simulink model "Demo_DSRC_BSM_I_and_II_Message_cs"  (Simulink 7.6)
settings: Solver=ode5  SolverMode=SingleTasking  StartTime=0.0  StopTime=40  FixedStep=1/20  RelTol=1e-3
PreLoadFcn:
  | check_NUTS_defined;
  | 
  | assignin('base',['model_closed_' bdroot],false);
InitFcn:
  | PreScanExperimentInitFcn(bdroot)
StopFcn:
  | PreScanExperimentStopFcn(bdroot)
libraries: simulink x9, PreScanSimulinkLibrary x8, PreScanUsefulBlocks x5, simulink_extras x1
(part 3 of 3)

== system Demo_DSRC_BSM_I_and_II_Message_cs/Mazda_RX8_1/Radius and confidence computation/Limitations ==
  note: Values of radius and center point
      |   coordinates on a straight path segment
  R : Inport
  d_Phi : Inport  Port=2
  "[xp,yp]" : Inport  Port=3
  Compare To Constant : simulink/Logic and Bit Operations/Compare To Constant  SystemSampleTime=-1  relop=<=  const=K_PPPATHISSTRAIGHT_M  LogicOutDataTypeMode=boolean  ZeroCross=off
  Compare To Zero : simulink/Logic and Bit Operations/Compare To Zero  SystemSampleTime=-1  relop=~=  LogicOutDataTypeMode=boolean  ZeroCross=off
  Compare To Zero1 : simulink/Logic and Bit Operations/Compare To Zero  SystemSampleTime=-1  relop=>  LogicOutDataTypeMode=boolean  ZeroCross=off
  Constant : Constant  Value=K_PPPATHISSTRAIGHT_M
  Constant1 : Constant  Value=[0;0]
  Logical Operator : Logic  Inputs=3  AllPortsSameDT=off  OutDataTypeStr=boolean  SampleTime=GPS_sample_time
  Switch1 : Switch  Criteria=u2 > Threshold  Threshold=0.5  SampleTime=GPS_sample_time
  Switch2 : Switch  Criteria=u2 > Threshold  Threshold=0.5  SampleTime=GPS_sample_time
  Radius [m] : Outport
  Center point : Outport  Port=2
  wires:
  R/1 -> Compare To Constant/1, Switch1/1, Compare To Zero1/1
  Compare To Zero/1 -> Logical Operator/1
  Compare To Constant/1 -> Logical Operator/2
  Logical Operator/1 -> Switch1/2, Switch2/2
  Constant/1 -> Switch1/3
  "[xp,yp]"/1 -> Switch2/1
  Constant1/1 -> Switch2/3
  Switch2/1 -> Center point/1
  Switch1/1 -> Radius [m]/1
  Compare To Zero1/1 -> Logical Operator/3
  d_Phi/1 -> Compare To Zero/1

== system Demo_DSRC_BSM_I_and_II_Message_cs/Mazda_RX8_1/Radius and confidence computation/Previous reading ==
  note: Determines previous value of signals
  Lat_in [deg] : Inport
  Long_in [deg] : Inport  Port=2
  Heading_in [deg] : Inport  Port=3
  Alt_in [m] : Inport  Port=4
  Demux : Demux
  Mux : Mux
  Unit Delay : UnitDelay  SampleTime=-1
  Lat2 [deg] : Outport
  Long2 [deg] : Outport  Port=2
  Heading2 [deg] : Outport  Port=3
  Alt2 [m] : Outport  Port=4
  wires:
  Lat_in [deg]/1 -> Mux/1
  Long_in [deg]/1 -> Mux/2
  Mux/1 -> Unit Delay/1
  Unit Delay/1 -> Demux/1
  Demux/1 -> Lat2 [deg]/1
  Demux/2 -> Long2 [deg]/1
  Heading_in [deg]/1 -> Mux/3
  Alt_in [m]/1 -> Mux/4
  Demux/3 -> Heading2 [deg]/1
  Demux/4 -> Alt2 [m]/1

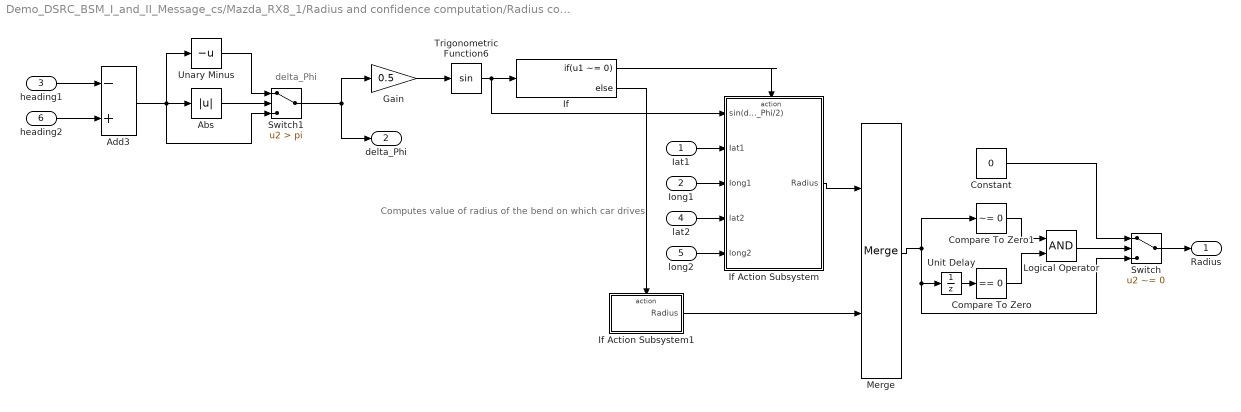
== system Demo_DSRC_BSM_I_and_II_Message_cs/Mazda_RX8_1/Radius and confidence computation/Radius computation ==
  note: delta_Phi
  note: Computes value of radius
      |    of the bend on which car drives
  Iat1 : Inport
  Iong1 : Inport  Port=2
  heading1 : Inport  Port=3
  lat2 : Inport  Port=4
  long2 : Inport  Port=5
  heading2 : Inport  Port=6
  Abs : Abs
  Add3 : Sum  Inputs=-+
  Compare To Zero : simulink/Logic and Bit Operations/Compare To Zero  SystemSampleTime=-1  relop===  LogicOutDataTypeMode=boolean  ZeroCross=off
  Compare To Zero1 : simulink/Logic and Bit Operations/Compare To Zero  SystemSampleTime=-1  relop=~=  LogicOutDataTypeMode=boolean  ZeroCross=off
  Constant : Constant  Value=0
  Gain : Gain  Gain=0.5
  If : If  IfExpression=u1 ~= 0
  If Action Subsystem : Subsystem  TreatAsAtomicUnit=on
  If Action Subsystem1 : Subsystem  TreatAsAtomicUnit=on
  Logical Operator : Logic  AllPortsSameDT=off  OutDataTypeStr=boolean
  Merge : Merge
  Switch : Switch  Criteria=u2 ~= 0  SampleTime=GPS_sample_time
  Switch1 : Switch  Criteria=u2 > Threshold  Threshold=pi
  Trigonometric Function6 : Trigonometry
  Unary Minus : UnaryMinus
  Unit Delay : UnitDelay  SampleTime=-1
  Radius : Outport
  delta_Phi : Outport  Port=2
  wires:
  Gain/1 -> Trigonometric Function6/1
  Trigonometric Function6/1 -> If/1, If Action Subsystem/1(sin(delta_Phi/2))
  If/1 -> If Action Subsystem/Action
  If/2 -> If Action Subsystem1/Action
  If Action Subsystem/1(Radius) -> Merge/1
  If Action Subsystem1/1(Radius) -> Merge/2
  Merge/1 -> Compare To Zero1/1, Unit Delay/1, Switch/3
  Unit Delay/1 -> Compare To Zero/1
  Compare To Zero1/1 -> Logical Operator/1
  Compare To Zero/1 -> Logical Operator/2
  Logical Operator/1 -> Switch/2
  Constant/1 -> Switch/1
  Switch/1 -> Radius/1
  heading1/1 -> Add3/1
  heading2/1 -> Add3/2
  Add3/1 -> Abs/1, Switch1/3, Unary Minus/1
  Abs/1 -> Switch1/2
  Unary Minus/1 -> Switch1/1
  Switch1/1 -> Gain/1, delta_Phi/1
  Iat1/1 -> If Action Subsystem/2(Iat1)
  Iong1/1 -> If Action Subsystem/3(Iong1)
  lat2/1 -> If Action Subsystem/4(lat2)
  long2/1 -> If Action Subsystem/5(long2)

== system Demo_DSRC_BSM_I_and_II_Message_cs/Mazda_RX8_1/Radius and confidence computation/Rate transition ==
  note: Changes rate transition of
      |    signals to GPS sampling rate
  Lat_in [deg] : Inport
  Long_in [deg] : Inport  Port=2
  Alt_in [m] : Inport  Port=3
  Heading_in [deg] : Inport  Port=4
  Demux : Demux
  Mux : Mux
  Rate Transition : RateTransition  Integrity=off  OutPortSampleTime=GPS_sample_time
  Lat [deg] : Outport
  Long [deg] : Outport  Port=2
  Heading [deg] : Outport  Port=3
  Alt [m] : Outport  Port=4
  wires:
  Lat_in [deg]/1 -> Mux/1
  Long_in [deg]/1 -> Mux/2
  Alt_in [m]/1 -> Mux/3
  Heading_in [deg]/1 -> Mux/4
  Mux/1 -> Rate Transition/1
  Rate Transition/1 -> Demux/1
  Demux/1 -> Lat [deg]/1
  Demux/2 -> Long [deg]/1
  Demux/3 -> Alt [m]/1
  Demux/4 -> Heading [deg]/1

== system Demo_DSRC_BSM_I_and_II_Message_cs/Mazda_RX8_1/SELF_Demux/compas converter ==
  rotz [rad] : Inport
  cart2compas : Subsystem
  rad2deg : Gain  Gain=180/pi
  heading [deg] : Outport
  wires:
  cart2compas/1(heading [deg]) -> heading [deg]/1
  rotz [rad]/1 -> rad2deg/1
  rad2deg/1 -> cart2compas/1(Angle [deg])

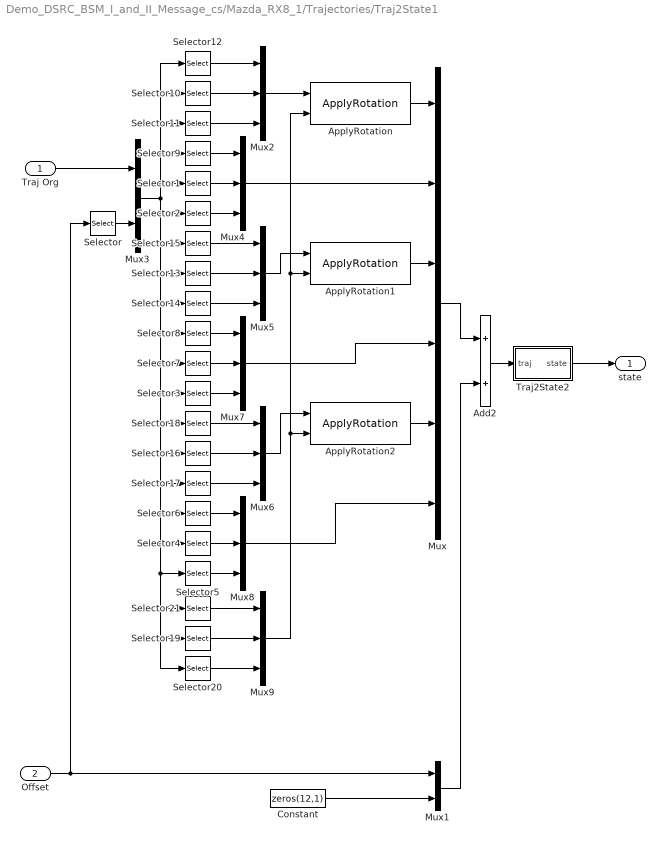
== system Demo_DSRC_BSM_I_and_II_Message_cs/Mazda_RX8_1/Trajectories/Traj2State1 ==
  Traj Org : Inport
  Offset : Inport  Port=2
  Add2 : Sum
  ApplyRotation : PreScanSimulinkLibrary/ApplyRotation  SystemSampleTime=-1
  ApplyRotation1 : PreScanSimulinkLibrary/ApplyRotation  SystemSampleTime=-1
  ApplyRotation2 : PreScanSimulinkLibrary/ApplyRotation  SystemSampleTime=-1
  Constant : Constant  Value=zeros(12,1)
  Mux : Mux  Inputs=6
  Mux1 : Mux  Inputs=2
  Mux{2,4..9} (7 alike) : Mux  Inputs=3
  Mux3 : Mux  Inputs=2
  Selector : Selector  InputPortWidth=6  IndexOptions=Index vector (dialog)  Indices=[4 5 6]  OutputSizes=1
  Selector1 : Selector  InputPortWidth=21  IndexOptions=Index vector (dialog)  Indices=[5]  OutputSizes=1
  Selector10 : Selector  InputPortWidth=21  IndexOptions=Index vector (dialog)  Indices=[2]  OutputSizes=1
  Selector11 : Selector  InputPortWidth=21  IndexOptions=Index vector (dialog)  Indices=[3]  OutputSizes=1
  Selector12 : Selector  InputPortWidth=21  IndexOptions=Index vector (dialog)  Indices=[1]  OutputSizes=1
  Selector13 : Selector  InputPortWidth=21  IndexOptions=Index vector (dialog)  Indices=[8]  OutputSizes=1
  Selector14 : Selector  InputPortWidth=21  IndexOptions=Index vector (dialog)  Indices=[9]  OutputSizes=1
  Selector15 : Selector  InputPortWidth=21  IndexOptions=Index vector (dialog)  Indices=[7]  OutputSizes=1
  Selector16 : Selector  InputPortWidth=21  IndexOptions=Index vector (dialog)  Indices=[14]  OutputSizes=1
  Selector17 : Selector  InputPortWidth=21  IndexOptions=Index vector (dialog)  Indices=[15]  OutputSizes=1
  Selector18 : Selector  InputPortWidth=21  IndexOptions=Index vector (dialog)  Indices=[13]  OutputSizes=1
  Selector19 : Selector  InputPortWidth=21  IndexOptions=Index vector (dialog)  Indices=[20]  OutputSizes=1
  Selector2 : Selector  InputPortWidth=21  IndexOptions=Index vector (dialog)  Indices=[6]  OutputSizes=1
  Selector20 : Selector  InputPortWidth=21  IndexOptions=Index vector (dialog)  Indices=[21]  OutputSizes=1
  Selector21 : Selector  InputPortWidth=21  IndexOptions=Index vector (dialog)  Indices=[19]  OutputSizes=1
  Selector3 : Selector  InputPortWidth=21  IndexOptions=Index vector (dialog)  Indices=[12]  OutputSizes=1
  Selector4 : Selector  InputPortWidth=21  IndexOptions=Index vector (dialog)  Indices=[17]  OutputSizes=1
  Selector5 : Selector  InputPortWidth=21  IndexOptions=Index vector (dialog)  Indices=[18]  OutputSizes=1
  Selector6 : Selector  InputPortWidth=21  IndexOptions=Index vector (dialog)  Indices=[16]  OutputSizes=1
  Selector7 : Selector  InputPortWidth=21  IndexOptions=Index vector (dialog)  Indices=[11]  OutputSizes=1
  Selector8 : Selector  InputPortWidth=21  IndexOptions=Index vector (dialog)  Indices=[10]  OutputSizes=1
  Selector9 : Selector  InputPortWidth=21  IndexOptions=Index vector (dialog)  Indices=[4]  OutputSizes=1
  Traj2State2 : Subsystem
  state : Outport
  wires:
  Mux9/1 -> ApplyRotation2/2, ApplyRotation1/2, ApplyRotation/2
  Selector20/1 -> Mux9/3
  Selector19/1 -> Mux9/2
  Selector21/1 -> Mux9/1
  Selector5/1 -> Mux8/3
  Selector4/1 -> Mux8/2
  Selector6/1 -> Mux8/1
  Mux8/1 -> Mux/6
  Mux6/1 -> ApplyRotation2/1
  Mux7/1 -> Mux/4
  ApplyRotation2/1 -> Mux/5
  Selector3/1 -> Mux7/3
  Selector7/1 -> Mux7/2
  Selector8/1 -> Mux7/1
  Mux4/1 -> Mux/2
  Mux5/1 -> ApplyRotation1/1
  ApplyRotation1/1 -> Mux/3
  Mux2/1 -> ApplyRotation/1
  ApplyRotation/1 -> Mux/1
  Selector2/1 -> Mux4/3
  Selector1/1 -> Mux4/2
  Selector9/1 -> Mux4/1
  Selector17/1 -> Mux6/3
  Selector16/1 -> Mux6/2
  Selector18/1 -> Mux6/1
  Selector14/1 -> Mux5/3
  Selector13/1 -> Mux5/2
  Selector15/1 -> Mux5/1
  Selector11/1 -> Mux2/3
  Selector10/1 -> Mux2/2
  Selector12/1 -> Mux2/1
  Mux3/1 -> Selector8/1, Selector7/1, Selector3/1, Selector18/1, Selector16/1, Selector17/1, Selector6/1, Selector20/1, Selector19/1, Selector21/1, Selector5/1, Selector4/1, Selector14/1, Selector13/1, Selector15/1, Selector2/1, Selector1/1, Selector9/1, Selector12/1, Selector10/1, Selector11/1
  Mux1/1 -> Add2/2
  Constant/1 -> Mux1/2
  Add2/1 -> Traj2State2/1(traj)
  Selector/1 -> Mux3/2
  Traj Org/1 -> Mux3/1
  Offset/1 -> Mux1/1, Selector/1
  Mux/1 -> Add2/1
  Traj2State2/1(state) -> state/1

== system Demo_DSRC_BSM_I_and_II_Message_cs/Mazda_RX8_1/Trajectories/Trajectory_1 ==
  From Workspace : FromWorkspace  VariableName=trajectory  SampleTime=TimeStep  OutputAfterFinalValue=Holding final value
  From Workspace1 : FromWorkspace  VariableName=trajectory  SampleTime=TimeStep  OutputAfterFinalValue=Setting to zero
  Mux : Mux  Inputs=2
  Selector1 : Selector  InputPortWidth=24  IndexOptions=Index vector (dialog)  Indices=[7:18]  OutputSizes=1
  Selector9 : Selector  InputPortWidth=24  IndexOptions=Index vector (dialog)  Indices=[1:6]  OutputSizes=1
  trajectory : Outport
  wires:
  Selector1/1 -> Mux/2
  Selector9/1 -> Mux/1
  Mux/1 -> trajectory/1
  From Workspace1/1 -> Selector1/1
  From Workspace/1 -> Selector9/1

== system Demo_DSRC_BSM_I_and_II_Message_cs/Ford_Fiesta_1/DSRC Receiver BSM I and II/DSRC_Rx_Demux/Reorder ==
  In : Inport
  Selector1 : Selector  InputPortWidth=InputPortWidth  IndexOptions=Index vector (dialog)  Indices=Elements  OutputSizes=1
  Out : Outport
  wires:
  In/1 -> Selector1/1
  Selector1/1 -> Out/1

== system Demo_DSRC_BSM_I_and_II_Message_cs/Ford_Fiesta_1/DSRC Receiver BSM I and II/DSRC_Rx_Demux/compas converter ==
  rotz [rad] : Inport
  cart2compas : Subsystem
  rad2deg : Gain  Gain=180/pi
  heading [deg] : Outport
  wires:
  cart2compas/1(heading [deg]) -> heading [deg]/1
  rotz [rad]/1 -> rad2deg/1
  rad2deg/1 -> cart2compas/1(Angle [deg])

== system Demo_DSRC_BSM_I_and_II_Message_cs/Ford_Fiesta_1/SELF_Demux/compas converter/cart2compas ==
  Angle [deg] : Inport
  Constant : Constant  Value=90
  Constant1 : Constant  Value=360
  Gain : Gain  Gain=1/360
  Gain1 : Gain  Gain=360
  Gain2 : Gain  Gain=-1
  Rounding Function : Rounding
  Sum : Sum  Inputs=|-+
  Sum1 : Sum  Inputs=-+|
  Sum2 : Sum  Inputs=++|
  heading [deg] : Outport
  wires:
  Sum2/1 -> heading [deg]/1
  Constant1/1 -> Sum2/1
  Gain2/1 -> Sum2/2
  Constant/1 -> Sum1/1
  Sum1/1 -> Sum/2, Gain/1
  Sum/1 -> Gain2/1
  Angle [deg]/1 -> Sum1/2
  Gain1/1 -> Sum/1
  Rounding Function/1 -> Gain1/1
  Gain/1 -> Rounding Function/1

== system Demo_DSRC_BSM_I_and_II_Message_cs/Ford_Fiesta_1/Trajectories/Traj2State1/Traj2State2 ==
  traj : Inport
  MuxState : Subsystem
  Traj2MuxState_Ext : Subsystem
  state : Outport
  wires:
  Traj2MuxState_Ext/9(Y [rad]) -> MuxState/9(Y [rad])
  Traj2MuxState_Ext/8(P [rad]) -> MuxState/8(P [rad])
  Traj2MuxState_Ext/7(R [rad]) -> MuxState/7(R [rad])
  Traj2MuxState_Ext/6(dz [m/s]) -> MuxState/6(dz [m/s])
  Traj2MuxState_Ext/5(dy [m/s]) -> MuxState/5(dy [m/s])
  Traj2MuxState_Ext/4(dx [m/s]) -> MuxState/4(dx [m/s])
  Traj2MuxState_Ext/3(z [m]) -> MuxState/3(z [m])
  Traj2MuxState_Ext/2(y [m]) -> MuxState/2(y [m])
  Traj2MuxState_Ext/1(x [m]) -> MuxState/1(x [m])
  MuxState/1(state) -> state/1
  traj/1 -> Traj2MuxState_Ext/1(Traj)

== system Demo_DSRC_BSM_I_and_II_Message_cs/Mazda_RX8_1/Basic Safety Message II/Enabled Basic Safety Message I and II/Enabled Confidence ==
  In1 : Inport
  Enable : EnablePort  PropagateVarSize=During execution
  Out1 : Outport  OutputWhenDisabled=reset  InitialOutput=0
  wires:
  In1/1 -> Out1/1

== system Demo_DSRC_BSM_I_and_II_Message_cs/Mazda_RX8_1/Basic Safety Message II/Enabled Basic Safety Message I and II/Enabled Eventflag ==
  In1 : Inport
  Enable : EnablePort  PropagateVarSize=During execution
  Out1 : Outport  OutputWhenDisabled=reset  InitialOutput=0
  wires:
  In1/1 -> Out1/1

== system Demo_DSRC_BSM_I_and_II_Message_cs/Mazda_RX8_1/Basic Safety Message II/Enabled Basic Safety Message I and II/Enabled Exterior lights ==
  In1 : Inport
  Enable : EnablePort  PropagateVarSize=During execution
  Out1 : Outport  OutputWhenDisabled=reset  InitialOutput=0
  wires:
  In1/1 -> Out1/1

== system Demo_DSRC_BSM_I_and_II_Message_cs/Mazda_RX8_1/Basic Safety Message II/Enabled Basic Safety Message I and II/Enabled itemCnt ==
  In1 : Inport
  Enable : EnablePort  PropagateVarSize=During execution
  Out1 : Outport  OutputWhenDisabled=reset  InitialOutput=0
  wires:
  In1/1 -> Out1/1

== system Demo_DSRC_BSM_I_and_II_Message_cs/Mazda_RX8_1/Basic Safety Message II/Enabled Basic Safety Message I and II/Enabled radiusOfCurve ==
  In1 : Inport
  Enable : EnablePort  PropagateVarSize=During execution
  Out1 : Outport  OutputWhenDisabled=reset  InitialOutput=0
  wires:
  In1/1 -> Out1/1

== system Demo_DSRC_BSM_I_and_II_Message_cs/Mazda_RX8_1/Basic Safety Message II/Enabled Basic Safety Message I and II/Enabled Throttle position ==
  In1 : Inport
  Enable : EnablePort  PropagateVarSize=During execution
  Out1 : Outport  OutputWhenDisabled=reset  InitialOutput=0
  wires:
  In1/1 -> Out1/1

== system Demo_DSRC_BSM_I_and_II_Message_cs/Mazda_RX8_1/Basic Safety Message II/Enabled Basic Safety Message I and II/Enabled path history ==
  In1 : Inport
  Enable : EnablePort  PropagateVarSize=During execution
  Out1 : Outport  OutputWhenDisabled=reset  InitialOutput=0
  wires:
  In1/1 -> Out1/1

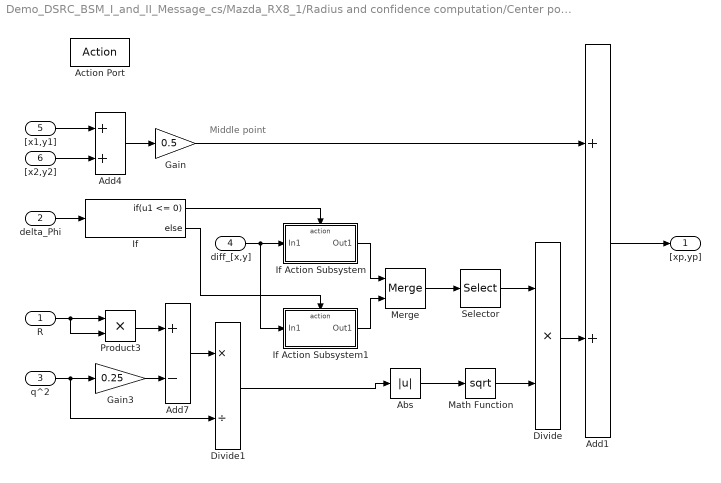
== system Demo_DSRC_BSM_I_and_II_Message_cs/Mazda_RX8_1/Radius and confidence computation/Center point of the bend/If Action Subsystem ==
  note: Middle point
  R : Inport
  delta_Phi : Inport  Port=2
  q^2 : Inport  Port=3
  diff_[x,y] : Inport  Port=4
  "[x1,y1]" : Inport  Port=5
  "[x2,y2]" : Inport  Port=6
  Action Port : ActionPort  PropagateVarSize=During execution  ActionType=then
  Abs : Abs
  Add1 : Sum
  Add4 : Sum
  Add7 : Sum  Inputs=+-
  Divide : Product  Inputs=**
  Divide1 : Product  Inputs=*/
  Gain : Gain  Gain=0.5
  Gain3 : Gain  Gain=0.25
  If : If  IfExpression=u1 <= 0
  If Action Subsystem : Subsystem  TreatAsAtomicUnit=on
  If Action Subsystem1 : Subsystem  TreatAsAtomicUnit=on
  Math Function : Math  Operator=sqrt  SaturateOnIntegerOverflow=on
  Merge : Merge
  Product3 : Product  RndMeth=Zero
  Selector : Selector  InputPortWidth=2  IndexOptions=Index vector (dialog)  Indices=[2 1]  OutputSizes=1
  "[xp,yp]" : Outport  InitialOutput=0
  wires:
  Add4/1 -> Gain/1
  "[x1,y1]"/1 -> Add4/1
  "[x2,y2]"/1 -> Add4/2
  delta_Phi/1 -> If/1
  If/1 -> If Action Subsystem/Action
  If/2 -> If Action Subsystem1/Action
  diff_[x,y]/1 -> If Action Subsystem/1(In1), If Action Subsystem1/1(In1)
  Gain3/1 -> Add7/2
  Product3/1 -> Add7/1
  Math Function/1 -> Divide/2
  If Action Subsystem/1(Out1) -> Merge/1
  If Action Subsystem1/1(Out1) -> Merge/2
  Merge/1 -> Selector/1
  q^2/1 -> Gain3/1, Divide1/2
  Selector/1 -> Divide/1
  Add1/1 -> "[xp,yp]"/1
  Divide/1 -> Add1/2
  Add7/1 -> Divide1/1
  Divide1/1 -> Abs/1
  R/1 -> Product3/1, Product3/2
  Gain/1 -> Add1/1
  Abs/1 -> Math Function/1

== system Demo_DSRC_BSM_I_and_II_Message_cs/Mazda_RX8_1/Radius and confidence computation/Center point of the bend/If Action Subsystem1 ==
  Action Port : ActionPort  PropagateVarSize=During execution  ActionType=else
  Constant : Constant  Value=zeros(2,1)
  "[xp,yp]" : Outport  InitialOutput=0
  wires:
  Constant/1 -> "[xp,yp]"/1

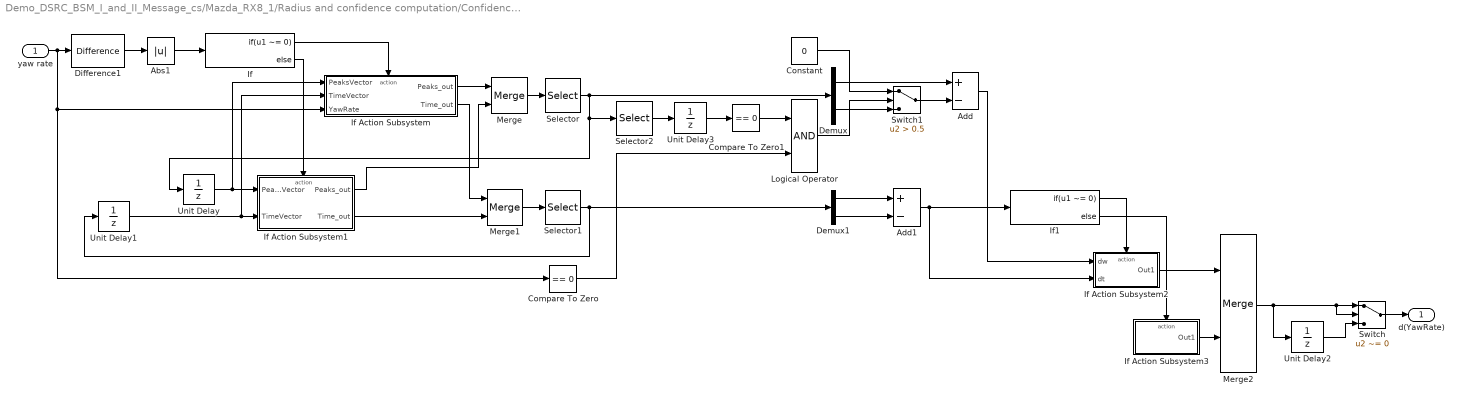
== system Demo_DSRC_BSM_I_and_II_Message_cs/Mazda_RX8_1/Radius and confidence computation/Confidence level/Derivative approximation ==
  yaw rate : Inport
  Abs1 : Abs
  Add : Sum  Inputs=+-
  Add1 : Sum  Inputs=+-
  Compare To Zero : simulink/Logic and Bit Operations/Compare To Zero  SystemSampleTime=-1  relop===  LogicOutDataTypeMode=uint8
  Compare To Zero1 : simulink/Logic and Bit Operations/Compare To Zero  SystemSampleTime=-1  relop===  LogicOutDataTypeMode=uint8
  Constant : Constant  Value=0
  Demux : Demux  Outputs=2
  Demux1 : Demux  Outputs=2
  Difference1 : simulink/Discrete/Difference  SystemSampleTime=-1  ICPrevInput=0.0  OutMin=[]  OutMax=[]  OutDataType=fixdt(1, 16)  OutScaling=2^-10  DoSatur=off
  If : If  IfExpression=u1 ~= 0
  If Action Subsystem : Subsystem  TreatAsAtomicUnit=on
  If Action Subsystem1 : Subsystem  TreatAsAtomicUnit=on
  If Action Subsystem2 : Subsystem  TreatAsAtomicUnit=on
  If Action Subsystem3 : Subsystem  TreatAsAtomicUnit=on
  If1 : If  IfExpression=u1 ~= 0
  Logical Operator : Logic  AllPortsSameDT=off  OutDataTypeStr=boolean
  Merge : Merge  InitialOutput=0
  Merge1 : Merge  InitialOutput=0
  Merge2 : Merge  InitialOutput=0
  Selector : Selector  InputPortWidth=3  IndexOptions=Index vector (dialog)  Indices=[1 2]  OutputSizes=1
  Selector1 : Selector  InputPortWidth=3  IndexOptions=Index vector (dialog)  Indices=[1 2]  OutputSizes=1
  Selector2 : Selector  InputPortWidth=2  IndexOptions=Index vector (dialog)  Indices=1  OutputSizes=1
  Switch : Switch  Criteria=u2 ~= 0  Threshold=1e-6
  Switch1 : Switch  Criteria=u2 > Threshold  Threshold=0.5
  Unit Delay{,1..3} (4 alike) : UnitDelay  SampleTime=-1
  d(YawRate) : Outport
  wires:
  If/1 -> If Action Subsystem/Action
  If/2 -> If Action Subsystem1/Action
  Unit Delay/1 -> If Action Subsystem1/1(PeaksVector), If Action Subsystem/1(PeaksVector)
  If Action Subsystem/1(Peaks_out) -> Merge/1
  Unit Delay1/1 -> If Action Subsystem1/2(TimeVector), If Action Subsystem/2(TimeVector)
  If Action Subsystem1/1(Peaks_out) -> Merge/2
  If Action Subsystem/2(Time_out) -> Merge1/1
  If Action Subsystem1/2(Time_out) -> Merge1/2
  Merge/1 -> Selector/1
  Merge1/1 -> Selector1/1
  Selector/1 -> Demux/1, Unit Delay/1, Selector2/1
  Selector1/1 -> Unit Delay1/1, Demux1/1
  Demux/1 -> Add/1
  Demux1/1 -> Add1/1
  Demux1/2 -> Add1/2
  Add/1 -> If Action Subsystem2/1(dw)
  Difference1/1 -> Abs1/1
  Merge2/1 -> Unit Delay2/1, Switch/1, Switch/2
  Unit Delay2/1 -> Switch/3
  Abs1/1 -> If/1
  Add1/1 -> If1/1, If Action Subsystem2/2(dt)
  If1/1 -> If Action Subsystem2/Action
  If1/2 -> If Action Subsystem3/Action
  If Action Subsystem2/1(Out1) -> Merge2/1
  If Action Subsystem3/1(Out1) -> Merge2/2
  yaw rate/1 -> Difference1/1, If Action Subsystem/3(YawRate), Compare To Zero/1
  Switch/1 -> d(YawRate)/1
  Selector2/1 -> Unit Delay3/1
  Unit Delay3/1 -> Compare To Zero1/1
  Compare To Zero1/1 -> Logical Operator/1
  Compare To Zero/1 -> Logical Operator/2
  Logical Operator/1 -> Switch1/2
  Demux/2 -> Switch1/3
  Switch1/1 -> Add/2
  Constant/1 -> Switch1/1

== system Demo_DSRC_BSM_I_and_II_Message_cs/Mazda_RX8_1/Radius and confidence computation/Confidence level/FIR filter1 ==
  In1 : Inport
  Add : Sum  Inputs=++++++++++
  Gain : Gain  Gain=0.1
  Unit Delay{1..9} (9 alike) : UnitDelay  SampleTime=-1
  Out1 : Outport
  wires:
  In1/1 -> Add/1, Unit Delay1/1
  Add/1 -> Gain/1
  Unit Delay1/1 -> Add/2, Unit Delay2/1
  Unit Delay2/1 -> Add/3, Unit Delay3/1
  Unit Delay3/1 -> Add/4, Unit Delay4/1
  Unit Delay4/1 -> Add/5, Unit Delay5/1
  Unit Delay5/1 -> Add/6, Unit Delay6/1
  Unit Delay6/1 -> Add/7, Unit Delay7/1
  Unit Delay7/1 -> Add/8, Unit Delay8/1
  Unit Delay8/1 -> Add/9, Unit Delay9/1
  Unit Delay9/1 -> Add/10
  Gain/1 -> Out1/1

== system Demo_DSRC_BSM_I_and_II_Message_cs/Mazda_RX8_1/Radius and confidence computation/Confidence level/FIR filter2 ==
  In1 : Inport
  Add : Sum  Inputs=++++++++
  Gain : Gain  Gain=1/8
  Unit Delay{1..7} (7 alike) : UnitDelay  SampleTime=-1
  Out1 : Outport
  wires:
  Unit Delay4/1 -> Add/5, Unit Delay5/1
  Unit Delay3/1 -> Unit Delay4/1, Add/4
  Unit Delay2/1 -> Unit Delay3/1, Add/3
  Unit Delay1/1 -> Unit Delay2/1, Add/2
  Add/1 -> Gain/1
  In1/1 -> Unit Delay1/1, Add/1
  Gain/1 -> Out1/1
  Unit Delay7/1 -> Add/8
  Unit Delay6/1 -> Add/7, Unit Delay7/1
  Unit Delay5/1 -> Add/6, Unit Delay6/1

== system Demo_DSRC_BSM_I_and_II_Message_cs/Mazda_RX8_1/Radius and confidence computation/Radius computation/If Action Subsystem ==
  sin(delta_Phi/2) : Inport
  Iat1 : Inport  Port=2
  Iong1 : Inport  Port=3
  lat2 : Inport  Port=4
  long2 : Inport  Port=5
  Action Port : ActionPort  PropagateVarSize=During execution  ActionType=then
  Abs : Abs
  Chord length1 : Subsystem
  Constant : Constant  Value=2
  Divide : Product  Inputs=*//
  Radius : Outport  InitialOutput=0
  wires:
  Constant/1 -> Divide/2
  Chord length1/1(chord) -> Divide/1
  sin(delta_Phi/2)/1 -> Divide/3
  Divide/1 -> Abs/1
  Abs/1 -> Radius/1
  Iong1/1 -> Chord length1/2(long1)
  long2/1 -> Chord length1/3(long2)
  Iat1/1 -> Chord length1/1(lat1)
  lat2/1 -> Chord length1/4(lat2)

== system Demo_DSRC_BSM_I_and_II_Message_cs/Mazda_RX8_1/Radius and confidence computation/Radius computation/If Action Subsystem1 ==
  Action Port : ActionPort  PropagateVarSize=During execution  ActionType=else
  Constant : Constant  Value=0
  Radius : Outport  InitialOutput=0
  wires:
  Constant/1 -> Radius/1

== system Demo_DSRC_BSM_I_and_II_Message_cs/Mazda_RX8_1/SELF_Demux/compas converter/cart2compas ==
  Angle [deg] : Inport
  Constant : Constant  Value=90
  Constant1 : Constant  Value=360
  Gain : Gain  Gain=1/360
  Gain1 : Gain  Gain=360
  Gain2 : Gain  Gain=-1
  Rounding Function : Rounding
  Sum : Sum  Inputs=|-+
  Sum1 : Sum  Inputs=-+|
  Sum2 : Sum  Inputs=++|
  heading [deg] : Outport
  wires:
  Sum2/1 -> heading [deg]/1
  Constant1/1 -> Sum2/1
  Gain2/1 -> Sum2/2
  Constant/1 -> Sum1/1
  Sum1/1 -> Sum/2, Gain/1
  Sum/1 -> Gain2/1
  Angle [deg]/1 -> Sum1/2
  Gain1/1 -> Sum/1
  Rounding Function/1 -> Gain1/1
  Gain/1 -> Rounding Function/1

== system Demo_DSRC_BSM_I_and_II_Message_cs/Mazda_RX8_1/Trajectories/Traj2State1/Traj2State2 ==
  traj : Inport
  MuxState : Subsystem
  Traj2MuxState_Ext : Subsystem
  state : Outport
  wires:
  Traj2MuxState_Ext/9(Y [rad]) -> MuxState/9(Y [rad])
  Traj2MuxState_Ext/8(P [rad]) -> MuxState/8(P [rad])
  Traj2MuxState_Ext/7(R [rad]) -> MuxState/7(R [rad])
  Traj2MuxState_Ext/6(dz [m/s]) -> MuxState/6(dz [m/s])
  Traj2MuxState_Ext/5(dy [m/s]) -> MuxState/5(dy [m/s])
  Traj2MuxState_Ext/4(dx [m/s]) -> MuxState/4(dx [m/s])
  Traj2MuxState_Ext/3(z [m]) -> MuxState/3(z [m])
  Traj2MuxState_Ext/2(y [m]) -> MuxState/2(y [m])
  Traj2MuxState_Ext/1(x [m]) -> MuxState/1(x [m])
  MuxState/1(state) -> state/1
  traj/1 -> Traj2MuxState_Ext/1(Traj)

== system Demo_DSRC_BSM_I_and_II_Message_cs/Ford_Fiesta_1/DSRC Receiver BSM I and II/DSRC_Rx_Demux/compas converter/cart2compas ==
  Angle [deg] : Inport
  Constant : Constant  Value=90
  Constant1 : Constant  Value=360
  Gain : Gain  Gain=1/360
  Gain1 : Gain  Gain=360
  Gain2 : Gain  Gain=-1
  Rounding Function : Rounding
  Sum : Sum  Inputs=|-+
  Sum1 : Sum  Inputs=-+|
  Sum2 : Sum  Inputs=++|
  heading [deg] : Outport
  wires:
  Sum2/1 -> heading [deg]/1
  Constant1/1 -> Sum2/1
  Gain2/1 -> Sum2/2
  Constant/1 -> Sum1/1
  Sum1/1 -> Sum/2, Gain/1
  Sum/1 -> Gain2/1
  Angle [deg]/1 -> Sum1/2
  Gain1/1 -> Sum/1
  Rounding Function/1 -> Gain1/1
  Gain/1 -> Rounding Function/1

== system Demo_DSRC_BSM_I_and_II_Message_cs/Ford_Fiesta_1/Trajectories/Traj2State1/Traj2State2/MuxState ==
  x [m] : Inport
  y [m] : Inport  Port=2
  z [m] : Inport  Port=3
  dx [m/s] : Inport  Port=4
  dy [m/s] : Inport  Port=5
  dz [m/s] : Inport  Port=6
  R [rad] : Inport  Port=7
  P [rad] : Inport  Port=8
  Y [rad] : Inport  Port=9
  Mux : Mux  Inputs=9
  state : Outport
  wires:
  z [m]/1 -> Mux/3
  y [m]/1 -> Mux/2
  x [m]/1 -> Mux/1
  Y [rad]/1 -> Mux/9
  P [rad]/1 -> Mux/8
  R [rad]/1 -> Mux/7
  dz [m/s]/1 -> Mux/6
  dy [m/s]/1 -> Mux/5
  dx [m/s]/1 -> Mux/4
  Mux/1 -> state/1

== system Demo_DSRC_BSM_I_and_II_Message_cs/Ford_Fiesta_1/Trajectories/Traj2State1/Traj2State2/Traj2MuxState_Ext ==
  Traj : Inport
  Terminator{1..9} (9 alike) : Terminator
  demux : Subsystem
  x [m] : Outport
  y [m] : Outport  Port=2
  z [m] : Outport  Port=3
  dx [m/s] : Outport  Port=4
  dy [m/s] : Outport  Port=5
  dz [m/s] : Outport  Port=6
  R [rad] : Outport  Port=7
  P [rad] : Outport  Port=8
  Y [rad] : Outport  Port=9
  wires:
  demux/9(Y) -> Y [rad]/1
  demux/7(R) -> R [rad]/1
  demux/5(vely) -> dy [m/s]/1
  demux/4(velx) -> dx [m/s]/1
  demux/10(velR) -> Terminator4/1
  demux/11(velP) -> Terminator5/1
  demux/12(velY) -> Terminator1/1
  demux/13(accx) -> Terminator8/1
  demux/14(accy) -> Terminator9/1
  demux/15(accz) -> Terminator7/1
  demux/18(accY) -> Terminator2/1
  demux/16(accR) -> Terminator3/1
  demux/17(accP) -> Terminator6/1
  demux/3(z) -> z [m]/1
  Traj/1 -> demux/1(traj)
  demux/6(velz) -> dz [m/s]/1
  demux/1(x) -> x [m]/1
  demux/2(y) -> y [m]/1
  demux/8(P) -> P [rad]/1

== system Demo_DSRC_BSM_I_and_II_Message_cs/Mazda_RX8_1/Radius and confidence computation/Center point of the bend/If Action Subsystem/If Action Subsystem ==
  In1 : Inport
  Action Port : ActionPort  PropagateVarSize=During execution  ActionType=then
  Gain1 : Gain  Gain=[1; -1]
  Out1 : Outport
  wires:
  In1/1 -> Gain1/1
  Gain1/1 -> Out1/1

== system Demo_DSRC_BSM_I_and_II_Message_cs/Mazda_RX8_1/Radius and confidence computation/Center point of the bend/If Action Subsystem/If Action Subsystem1 ==
  In1 : Inport
  Action Port : ActionPort  PropagateVarSize=During execution  ActionType=else
  Gain1 : Gain  Gain=[-1; 1]
  Out1 : Outport
  wires:
  In1/1 -> Gain1/1
  Gain1/1 -> Out1/1

== system Demo_DSRC_BSM_I_and_II_Message_cs/Mazda_RX8_1/Radius and confidence computation/Confidence level/Derivative approximation/If Action Subsystem ==
  PeaksVector : Inport
  TimeVector : Inport  Port=2
  YawRate : Inport  Port=3
  Action Port : ActionPort  PropagateVarSize=During execution  ActionType=then
  Demux : Demux  Outputs=2
  Demux1 : Demux  Outputs=2
  Digital Clock : DigitalClock  SampleTime=GPS_sample_time
  Mux : Mux  Inputs=3
  Mux1 : Mux  Inputs=3
  Peaks_out : Outport  InitialOutput=0
  Time_out : Outport  Port=2  InitialOutput=0
  wires:
  TimeVector/1 -> Demux/1
  Demux/1 -> Mux/2
  Digital Clock/1 -> Mux/1
  Mux/1 -> Time_out/1
  PeaksVector/1 -> Demux1/1
  Demux1/1 -> Mux1/2
  YawRate/1 -> Mux1/1
  Mux1/1 -> Peaks_out/1
  Demux/2 -> Mux/3
  Demux1/2 -> Mux1/3

== system Demo_DSRC_BSM_I_and_II_Message_cs/Mazda_RX8_1/Radius and confidence computation/Confidence level/Derivative approximation/If Action Subsystem1 ==
  PeaksVector : Inport
  TimeVector : Inport  Port=2
  Action Port : ActionPort  PropagateVarSize=During execution  ActionType=else
  Constant : Constant  Value=0
  Constant1 : Constant  Value=0
  Mux : Mux  Inputs=2
  Mux1 : Mux  Inputs=2
  Peaks_out : Outport  InitialOutput=0
  Time_out : Outport  Port=2  InitialOutput=0
  wires:
  PeaksVector/1 -> Mux/1
  Mux/1 -> Peaks_out/1
  Constant/1 -> Mux/2
  TimeVector/1 -> Mux1/1
  Constant1/1 -> Mux1/2
  Mux1/1 -> Time_out/1

== system Demo_DSRC_BSM_I_and_II_Message_cs/Mazda_RX8_1/Radius and confidence computation/Confidence level/Derivative approximation/If Action Subsystem2 ==
  dw : Inport
  dt : Inport  Port=2
  Action Port : ActionPort  PropagateVarSize=During execution  ActionType=then
  Divide : Product  Inputs=*/
  Out1 : Outport  InitialOutput=0
  wires:
  dw/1 -> Divide/1
  dt/1 -> Divide/2
  Divide/1 -> Out1/1

== system Demo_DSRC_BSM_I_and_II_Message_cs/Mazda_RX8_1/Radius and confidence computation/Confidence level/Derivative approximation/If Action Subsystem3 ==
  Action Port : ActionPort  PropagateVarSize=During execution  ActionType=else
  Constant : Constant  Value=0
  Out1 : Outport  InitialOutput=0
  wires:
  Constant/1 -> Out1/1

== system Demo_DSRC_BSM_I_and_II_Message_cs/Mazda_RX8_1/Radius and confidence computation/Radius computation/If Action Subsystem/Chord length1 ==
  note: Computes chord length from two GPS readings
  lat1 : Inport
  long1 : Inport  Port=2
  long2 : Inport  Port=3
  lat2 : Inport  Port=4
  Add1 : Sum  Inputs=+-
  Add2 : Sum
  Meridian Radius of Earth : Constant  Value=6367454
  Product : Product  RndMeth=Zero
  Product1 : Product  Inputs=3  RndMeth=Zero
  Product2 : Product  RndMeth=Zero
  Trigonometric Function : Trigonometry  Operator=acos
  Trigonometric Function1 : Trigonometry  Operator=cos
  Trigonometric Function2 : Trigonometry  Operator=cos
  Trigonometric Function3 : Trigonometry  Operator=cos
  Trigonometric Function4 : Trigonometry
  Trigonometric Function5 : Trigonometry
  chord : Outport
  wires:
  Meridian Radius of Earth/1 -> Product/1
  Trigonometric Function/1 -> Product/2
  Trigonometric Function1/1 -> Product1/1
  Trigonometric Function2/1 -> Product1/2
  lat1/1 -> Trigonometric Function1/1, Trigonometric Function4/1
  lat2/1 -> Trigonometric Function2/1, Trigonometric Function5/1
  Add1/1 -> Trigonometric Function3/1
  Trigonometric Function3/1 -> Product1/3
  Product1/1 -> Add2/1
  Trigonometric Function4/1 -> Product2/1
  Trigonometric Function5/1 -> Product2/2
  Product2/1 -> Add2/2
  Add2/1 -> Trigonometric Function/1
  long1/1 -> Add1/1
  Product/1 -> chord/1
  long2/1 -> Add1/2

== system Demo_DSRC_BSM_I_and_II_Message_cs/Mazda_RX8_1/Trajectories/Traj2State1/Traj2State2/MuxState ==
  x [m] : Inport
  y [m] : Inport  Port=2
  z [m] : Inport  Port=3
  dx [m/s] : Inport  Port=4
  dy [m/s] : Inport  Port=5
  dz [m/s] : Inport  Port=6
  R [rad] : Inport  Port=7
  P [rad] : Inport  Port=8
  Y [rad] : Inport  Port=9
  Mux : Mux  Inputs=9
  state : Outport
  wires:
  z [m]/1 -> Mux/3
  y [m]/1 -> Mux/2
  x [m]/1 -> Mux/1
  Y [rad]/1 -> Mux/9
  P [rad]/1 -> Mux/8
  R [rad]/1 -> Mux/7
  dz [m/s]/1 -> Mux/6
  dy [m/s]/1 -> Mux/5
  dx [m/s]/1 -> Mux/4
  Mux/1 -> state/1

== system Demo_DSRC_BSM_I_and_II_Message_cs/Mazda_RX8_1/Trajectories/Traj2State1/Traj2State2/Traj2MuxState_Ext ==
  Traj : Inport
  Terminator{1..9} (9 alike) : Terminator
  demux : Subsystem
  x [m] : Outport
  y [m] : Outport  Port=2
  z [m] : Outport  Port=3
  dx [m/s] : Outport  Port=4
  dy [m/s] : Outport  Port=5
  dz [m/s] : Outport  Port=6
  R [rad] : Outport  Port=7
  P [rad] : Outport  Port=8
  Y [rad] : Outport  Port=9
  wires:
  demux/9(Y) -> Y [rad]/1
  demux/7(R) -> R [rad]/1
  demux/5(vely) -> dy [m/s]/1
  demux/4(velx) -> dx [m/s]/1
  demux/10(velR) -> Terminator4/1
  demux/11(velP) -> Terminator5/1
  demux/12(velY) -> Terminator1/1
  demux/13(accx) -> Terminator8/1
  demux/14(accy) -> Terminator9/1
  demux/15(accz) -> Terminator7/1
  demux/18(accY) -> Terminator2/1
  demux/16(accR) -> Terminator3/1
  demux/17(accP) -> Terminator6/1
  demux/3(z) -> z [m]/1
  Traj/1 -> demux/1(traj)
  demux/6(velz) -> dz [m/s]/1
  demux/1(x) -> x [m]/1
  demux/2(y) -> y [m]/1
  demux/8(P) -> P [rad]/1

== system Demo_DSRC_BSM_I_and_II_Message_cs/Ford_Fiesta_1/Trajectories/Traj2State1/Traj2State2/Traj2MuxState_Ext/demux ==
  traj : Inport
  Demux : Demux  Outputs=18
  x : Outport
  y : Outport  Port=2
  z : Outport  Port=3
  velx : Outport  Port=4
  vely : Outport  Port=5
  velz : Outport  Port=6
  R : Outport  Port=7
  P : Outport  Port=8
  Y : Outport  Port=9
  velR : Outport  Port=10
  velP : Outport  Port=11
  velY : Outport  Port=12
  accx : Outport  Port=13
  accy : Outport  Port=14
  accz : Outport  Port=15
  accR : Outport  Port=16
  accP : Outport  Port=17
  accY : Outport  Port=18
  wires:
  Demux/18 -> accY/1
  Demux/17 -> accP/1
  Demux/16 -> accR/1
  Demux/15 -> accz/1
  Demux/14 -> accy/1
  Demux/13 -> accx/1
  Demux/12 -> velY/1
  Demux/11 -> velP/1
  Demux/10 -> velR/1
  Demux/9 -> velz/1
  Demux/8 -> vely/1
  Demux/7 -> velx/1
  Demux/6 -> Y/1
  Demux/5 -> P/1
  traj/1 -> Demux/1
  Demux/4 -> R/1
  Demux/3 -> z/1
  Demux/2 -> y/1
  Demux/1 -> x/1

== system Demo_DSRC_BSM_I_and_II_Message_cs/Mazda_RX8_1/Trajectories/Traj2State1/Traj2State2/Traj2MuxState_Ext/demux ==
  traj : Inport
  Demux : Demux  Outputs=18
  x : Outport
  y : Outport  Port=2
  z : Outport  Port=3
  velx : Outport  Port=4
  vely : Outport  Port=5
  velz : Outport  Port=6
  R : Outport  Port=7
  P : Outport  Port=8
  Y : Outport  Port=9
  velR : Outport  Port=10
  velP : Outport  Port=11
  velY : Outport  Port=12
  accx : Outport  Port=13
  accy : Outport  Port=14
  accz : Outport  Port=15
  accR : Outport  Port=16
  accP : Outport  Port=17
  accY : Outport  Port=18
  wires:
  Demux/18 -> accY/1
  Demux/17 -> accP/1
  Demux/16 -> accR/1
  Demux/15 -> accz/1
  Demux/14 -> accy/1
  Demux/13 -> accx/1
  Demux/12 -> velY/1
  Demux/11 -> velP/1
  Demux/10 -> velR/1
  Demux/9 -> velz/1
  Demux/8 -> vely/1
  Demux/7 -> velx/1
  Demux/6 -> Y/1
  Demux/5 -> P/1
  traj/1 -> Demux/1
  Demux/4 -> R/1
  Demux/3 -> z/1
  Demux/2 -> y/1
  Demux/1 -> x/1

== matlab function Mazda_RX8_1/J2735 Encoder Basic Safety Message I and II/Embedded MATLAB Function ==
  data: u1 input double; y output double; u2 input double; u3 input double; u4 input double; u5 input double; u6 input double; u7 input double; u8 input double; u9 input double; u10 input double; u11 input double; u12 input double; u13 input double; u14 input double; u15 input double; u16 input double; u17 input double; u18 input double; u19 input double; u20 input double; u21 input double; u22 input double; u23 input double; u24 input double; u25 input double; u26 input double; u27 input double; u28 input double; u29 input double; u30 input double; u31 input double; u32 input double; u33 input double; u34 input double; u35 input double; u36 input double; u37 input double; u38 input double; u39 input double; u40 input double; u41 input double; u42 input double; u43 input double; u44 input double; u45 input double; u46 input double; u47 input double; u48 input double; u49 input double; u50 input double; u51 input double; u52 input double; u53 input double; u54 input double; u55 input double; u56 input double; u57 input double; u58 input double; u59 input double; u60 input double; u61 input double; u62 input double; u63 input double
function y = fcn(u1,u2,u3,u4,u5,u6,u7,u8,u9,u10,u11,u12,u13,u14,u15,u16,u17,u18,u19,u20,u21,u22,u23,u24,u25,u26,u27,u28,u29,u30,u31,u32,u33,u34,u35,u36,u37,u38,u39,u40,u41,u42,u43,u44,u45,u46,u47,u48,u49,u50,u51,u52,u53,u54,u55,u56,u57,u58,u59,u60,u61,u62,u63)
%#eml
y = zeros(1,63,'double');
y(1) = u1;
y(2) = u2;
y(3) = u3;
y(4) = u4;
y(5) = u5;
y(6) = u6;
y(7) = u7;
y(8) = u8;
y(9) = u9;
y(10) = u10;
y(11) = u11;
y(12) = u12;
y(13) = u13;
y(14) = u14;
y(15) = u15;
y(16) = u16;
y(17) = u17;
y(18) = u18;
y(19) = u19;
y(20) = u20;
y(21) = u21;
y(22) = u22;
y(23) = u23;
y(24) = u24;
y(25) = u25;
y(26) = u26;
y(27) = u27;
y(28) = u28;
y(29) = u29;
y(30) = u30;
y(31) = u31;
y(32) = u32;
y(33) = u33;
y(34) = u34;
y(35) = u35;
y(36) = u36;
y(37) = u37;
y(38) = u38;
y(39) = u39;
y(40) = u40;
y(41) = u41;
y(42) = u42;
y(43) = u43;
y(44) = u44;
y(45) = u45;
y(46) = u46;
y(47) = u47;
y(48) = u48;
y(49) = u49;
y(50) = u50;
y(51) = u51;
y(52) = u52;
y(53) = u53;
y(54) = u54;
y(55) = u55;
y(56) = u56;
y(57) = u57;
y(58) = u58;
y(59) = u59;
y(60) = u60;
y(61) = u61;
y(62) = u62;
y(63) = u63;

== matlab function Mazda_RX8_1/Basic Safety Message II/BSM-II Unpacker/Embedded MATLAB Function ==
  data: u input double; y output double
function y = fcn(u)
%#eml
r = zeros(37,1,'double');
for i=1:36
    r(i) = r(i) + double(u((i*5)-4));
    r(i) = r(i) + double(u((i*5)-3))/1000;
    r(i) = r(i) + double(u((i*5)-2))/1000000;
    r(i) = r(i) + double(u((i*5)-1))/1000000000;
    r(i) = r(i) + double(u((i*5)))/1000000000000;
end
    r(37) = r(37) + double(u(181));
    r(37) = r(37) + double(u(182))/1000;
    r(37) = r(37) + double(u(183))/1000000;
    r(37) = r(37) + double(u(184))/1000000000;
y = r;

== matlab function Ford_Fiesta_1/Unpack Enable Descriptor/Create enabled bitvector ==
  data: inp input double; bitvector output double
function bitvector = DoubleToBits(inp)
%#eml
%eml.extrinsic('dec2bin');
%binchars = dec2bin(u,8);
%doedah = binchars(1);
r = zeros(7,1);
left = round(inp);
if left > 63
    left = left - 64;
    r(1) = 1;
end
if left > 31
    left = left - 32;
    r(2) = 1;
end
if left > 15
    left = left - 16;
    r(3) = 1;
end
if left > 7
    left = left - 8;
    r(4) = 1;
end
if left > 3
    left = left - 4;
    r(5) = 1;
end
if left > 1
    left = left - 2;
    r(6) = 1;
end
if left > 0
    left = left - 1;
    r(7) = 1;
end
bitvector = r;

== matlab function Mazda_RX8_1/Basic Safety Message II/Enabled Basic Safety Message I and II/Create enabled bitvector ==
  data: inp input double; bitvector output double
function bitvector = DoubleToBits(inp)
%#eml
%eml.extrinsic('dec2bin');
%binchars = dec2bin(u,8);
%doedah = binchars(1);
r = zeros(7,1);
left = round(inp);
if left > 63
    left = left - 64;
    r(1) = 1;
end
if left > 31
    left = left - 32;
    r(2) = 1;
end
if left > 15
    left = left - 16;
    r(3) = 1;
end
if left > 7
    left = left - 8;
    r(4) = 1;
end
if left > 3
    left = left - 4;
    r(5) = 1;
end
if left > 1
    left = left - 2;
    r(6) = 1;
end
if left > 0
    left = left - 1;
    r(7) = 1;
end
bitvector = r;

== matlab function Mazda_RX8_1/Basic Safety Message II/Enabled Basic Safety Message I and II/FindDescriptor ==
  data: u input double; y output double; itOut output double; itIn input double
function [y,itOut]= fcn(u,itIn)
%#eml
y=u(itIn);
itOut = itIn + 1;
if itOut > 10
    itOut = 1;
end
end

== matlab function Ford_Fiesta_1/J2735 Decoder Basic Safety Message I and II/Embedded MATLAB Function ==
  data: u input double; y output double
function y = fcn(u)

r = zeros(184,1,'uint8');
for i=1:36
    r((i*5)-4)= uint8(u(i));
    l = double(u(i)) - double(r((i*5)-4));
    
    r((i*5)-3)= uint8(l*1000);
    l = double((l * 1000)) - double(r((i*5)-3));
    
    r((i*5)-2) = uint8(l*1000);
    l = double((l * 1000)) - double(r((i*5)-2));
    
    r((i*5)-1) = uint8(l*1000);
    l = double((l * 1000)) - double(r((i*5)-1));
    
    r((i*5)) = uint8(l*1000);
    l = double((l * 1000)) - double(r((i*5)));
    
end
    i=37;
    r((i*5)-4)= uint8(u(i));
    l = double(u(i)) - double(r((i*5)-4));
    
    r((i*5)-3)= uint8(l*1000);
    l = double((l * 1000)) - double(r((i*5)-3));
    
    r((i*5)-2) = uint8(l*1000);
    l = double((l * 1000)) - double(r((i*5)-2));
    
    r((i*5)-1) = uint8(l*1000);
    l = double((l * 1000)) - double(r((i*5)-1));

y = r;
